simulink model "S250205simul_switch_2023a"  (R2024b)
settings: Solver=FixedStepDiscrete  StartTime=0  StopTime=60  FixedStep=0.01  RelTol=1e-3  AbsTol=1e-6
undefined symbols (not defined in the file or in its folder): a, b, c, d, f, g, switch_logic, VmcRgn_C_C, VmcRgn_J_C, VmcRgn_k_1to2_C, VmcRgn_k_2to3_C, VmcRgn_k_2to6_C, VmcRgn_k_3to4_C, VmcRgn_k_5to2_C, VmcRgn_k_6to2_C, VmcRgn_Kp_C, VmcRgn_L_C, VmcRgn_lf_C, VmcRgn_lr_C, VmcRgn_mass_C, VmcRgn_Mot2Whl_C, VmcRgn_PedDep_thrs_C, VmcRgn_phs2_k_C, VmcRgn_phs2_tq_C, VmcRgn_phs3_tq_C, VmcRgn_phs4_tq_C, VmcRgn_phs5_tq_C, VmcRgn_phs6_tq_C, VmcRgn_r_e_C, VmcRgn_R_whl_C, VmcRgn_SAS_thrs_C, VmcRgn_slip_max_C, VmcRgn_slip_max_gain_F_C, VmcRgn_slip_max_gain_R_C, VmcRgn_sup_tq_C, VmcRgn_t_pred_C, VmcRgn_target_w_acc_C, VmcRgn_tTs, VmcRgn_tTsinMs_C, VmcRgn_Yaw_thrs_C, yaw_flag
libraries: simulink x26, simulink_need_slupdate x1
(part 3 of 3)

== system S250205simul_switch_2023a/SlipCtrlFL/DiscreteDerivative ==
  note: U(k)
  note: ( U(k) - U(k-1) )
  U : Inport
  Constant : Constant  Value=Ts  OutDataTypeStr=uint16
  Data Type Conversion : DataTypeConversion  OutDataTypeStr=single  SaturateOnIntegerOverflow=off  RndMeth=Floor
  Data Type Conversion1 : DataTypeConversion  OutDataTypeStr=single  SaturateOnIntegerOverflow=off  RndMeth=Floor
  Data Type Conversion2 : DataTypeConversion  RndMeth=Round  LockScale=on
  Diff : Sum  Description=Add in CPU  Inputs=+-  OutDataTypeStr=single  AccumDataTypeStr=single  SaturateOnIntegerOverflow=on
  Divide : Product  Inputs=*/  OutDataTypeStr=single
  UD : UnitDelay  Description=Store in Global RAM  DisableCoverage=on  SampleTime=-1  HasFrameUpgradeWarning=on
  ms-to-s : Gain  Gain=0.001  ParamDataTypeStr=single  OutDataTypeStr=single
  Y : Outport  OutDataTypeStr=out_type  InitialOutput=0  VectorParamsAs1DForOutWhenUnconnected=off
  wires:
  Constant/1 -> Data Type Conversion1/1
  Divide/1 -> Diff/1, UD/1
  Diff/1 -> Data Type Conversion2/1
  UD/1 -> Diff/2  "U(k-1)"
  U/1 -> Data Type Conversion/1
  Data Type Conversion/1 -> Divide/1
  Data Type Conversion1/1 -> ms-to-s/1
  ms-to-s/1 -> Divide/2
  Data Type Conversion2/1 -> Y/1

== system S250205simul_switch_2023a/SlipCtrlFL/Sat_-1to1 ==
  In1 : Inport
  Constant : Constant  Value=-1  OutDataTypeStr=single
  Constant1 : Constant  OutDataTypeStr=single
  Switch1 : Switch  Criteria=u2 > Threshold  Threshold=1  SaturateOnIntegerOverflow=off  InputSameDT=off
  Switch4 : Switch  Criteria=u2 > Threshold  Threshold=-1  SaturateOnIntegerOverflow=off  InputSameDT=off
  Out1 : Outport
  wires:
  In1/1 -> Switch4/1, Switch4/2
  Switch4/1 -> Switch1/3, Switch1/2
  Constant/1 -> Switch4/3
  Constant1/1 -> Switch1/1
  Switch1/1 -> Out1/1

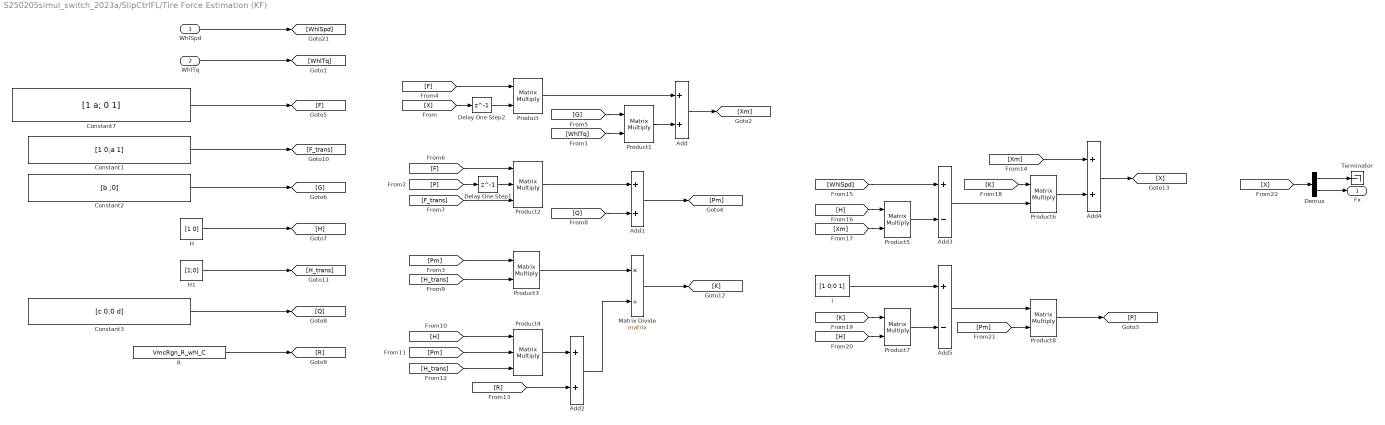
== system S250205simul_switch_2023a/SlipCtrlFL/Tire Force Estimation (KF) ==
  WhlSpd : Inport
  WhlTq : Inport  Port=2
  Add : Sum  OutDataTypeStr=single
  Add1 : Sum  OutDataTypeStr=single
  Add2 : Sum
  Add3 : Sum  Inputs=+-  OutDataTypeStr=single
  Add4 : Sum  OutDataTypeStr=single
  Add5 : Sum  Inputs=+-  OutDataTypeStr=single
  Constant1 : Constant  Value=[1 0;a 1]  VectorParams1D=off  SampleTime=-1  LockScale=on  mask(Customized constant block){}
      settings: AttributesFormatString=OutType: %<OutDataTypeStr>
  Constant2 : Constant  Value=[b ;0]  VectorParams1D=off  SampleTime=-1  LockScale=on  mask(Customized constant block){}
      settings: AttributesFormatString=OutType: %<OutDataTypeStr>
  Constant3 : Constant  Value=[c 0;0 d]  VectorParams1D=off  SampleTime=-1  LockScale=on  mask(Customized constant block){}
      settings: AttributesFormatString=OutType: %<OutDataTypeStr>
  Constant7 : Constant  Value=[1 a; 0 1]  VectorParams1D=off  SampleTime=-1  LockScale=on  mask(Customized constant block){}
      settings: AttributesFormatString=OutType: %<OutDataTypeStr>
  Delay One Step1 : Delay  DelayLength=1  InitialCondition=diag([64.1 0])
  Delay One Step2 : Delay  DelayLength=1  InitialCondition=[64.1; 0]
  Demux : Demux  Outputs=2
  H : Constant  Value=[1 0]  VectorParams1D=off  OutDataTypeStr=single  SampleTime=-1
  H1 : Constant  Value=[1;0]  VectorParams1D=off  OutDataTypeStr=single  SampleTime=-1
  I : Constant  Value=[1 0;0 1]  VectorParams1D=off  OutDataTypeStr=single  SampleTime=-1
  Matrix Divide : Product  Inputs=*/  Multiplication=Matrix(*)  OutDataTypeStr=single
  Product{,1,3,5..8} (7 alike) : Product  Multiplication=Matrix(*)
  Product2 : Product  Inputs=3  Multiplication=Matrix(*)
  Product4 : Product  Inputs=3  Multiplication=Matrix(*)
  R : Constant  Value=VmcRgn_R_whl_C  VectorParams1D=off  OutDataTypeStr=single  SampleTime=-1
  Terminator : Terminator
  Fx : Outport
  wires:
  WhlSpd/1 -> [WhlSpd]
  WhlTq/1 -> [WhlTq]
  [F] -> Product/1
  Product/1 -> Add/1
  [G] -> Product1/1
  [WhlTq] -> Product1/2
  Product1/1 -> Add/2
  Add/1 -> [Xm]
  [P] -> Delay One Step1/1
  Delay One Step1/1 -> Product2/2
  [F_trans] -> Product2/3
  Add1/1 -> [Pm]
  [Pm] -> Product3/1
  Constant7/1 -> [F]
  Constant2/1 -> [G]
  H/1 -> [H]
  Constant3/1 -> [Q]
  R/1 -> [R]
  [F] -> Product2/1
  Constant1/1 -> [F_trans]
  H1/1 -> [H_trans]
  Product2/1 -> Add1/1
  [Q] -> Add1/2
  [H_trans] -> Product3/2
  [H] -> Product4/1
  [H_trans] -> Product4/3
  [Pm] -> Product4/2
  Product4/1 -> Add2/1
  [R] -> Add2/2
  Product3/1 -> Matrix Divide/1
  Add2/1 -> Matrix Divide/2
  Matrix Divide/1 -> [K]
  [WhlSpd] -> Add3/1
  Product5/1 -> Add3/2
  [H] -> Product5/1
  [Xm] -> Product5/2
  Add3/1 -> Product6/2
  [K] -> Product6/1
  Product6/1 -> Add4/2
  [Xm] -> Add4/1
  Add4/1 -> [X]
  I/1 -> Add5/1
  [K] -> Product7/1
  [H] -> Product7/2
  Product7/1 -> Add5/2
  Add5/1 -> Product8/1
  [Pm] -> Product8/2
  Product8/1 -> [P]
  Delay One Step2/1 -> Product/2
  [X] -> Delay One Step2/1
  Demux/2 -> Fx/1
  Demux/1 -> Terminator/1
  [X] -> Demux/1

== system S250205simul_switch_2023a/SlipCtrlFL/Triggered Subsystem ==
  In1 : Inport
  Trigger : TriggerPort  VariantControl=(inherit)
  Out1 : Outport
  wires:
  In1/1 -> Out1/1

== system S250205simul_switch_2023a/SlipCtrlFR/DiscreteDerivative ==
  note: U(k)
  note: ( U(k) - U(k-1) )
  U : Inport
  Constant : Constant  Value=Ts  OutDataTypeStr=uint16
  Data Type Conversion : DataTypeConversion  OutDataTypeStr=single  SaturateOnIntegerOverflow=off  RndMeth=Floor
  Data Type Conversion1 : DataTypeConversion  OutDataTypeStr=single  SaturateOnIntegerOverflow=off  RndMeth=Floor
  Data Type Conversion2 : DataTypeConversion  RndMeth=Round  LockScale=on
  Diff : Sum  Description=Add in CPU  Inputs=+-  OutDataTypeStr=single  AccumDataTypeStr=single  SaturateOnIntegerOverflow=on
  Divide : Product  Inputs=*/  OutDataTypeStr=single
  UD : UnitDelay  Description=Store in Global RAM  DisableCoverage=on  SampleTime=-1  HasFrameUpgradeWarning=on
  ms-to-s : Gain  Gain=0.001  ParamDataTypeStr=single  OutDataTypeStr=single
  Y : Outport  OutDataTypeStr=out_type  InitialOutput=0  VectorParamsAs1DForOutWhenUnconnected=off
  wires:
  Constant/1 -> Data Type Conversion1/1
  Divide/1 -> Diff/1, UD/1
  Diff/1 -> Data Type Conversion2/1
  UD/1 -> Diff/2  "U(k-1)"
  U/1 -> Data Type Conversion/1
  Data Type Conversion/1 -> Divide/1
  Data Type Conversion1/1 -> ms-to-s/1
  ms-to-s/1 -> Divide/2
  Data Type Conversion2/1 -> Y/1

== system S250205simul_switch_2023a/SlipCtrlFR/Sat_-1to1 ==
  In1 : Inport
  Constant : Constant  Value=-1  OutDataTypeStr=single
  Constant1 : Constant  OutDataTypeStr=single
  Switch1 : Switch  Criteria=u2 > Threshold  Threshold=1  SaturateOnIntegerOverflow=off  InputSameDT=off
  Switch4 : Switch  Criteria=u2 > Threshold  Threshold=-1  SaturateOnIntegerOverflow=off  InputSameDT=off
  Out1 : Outport
  wires:
  In1/1 -> Switch4/1, Switch4/2
  Switch4/1 -> Switch1/3, Switch1/2
  Constant/1 -> Switch4/3
  Constant1/1 -> Switch1/1
  Switch1/1 -> Out1/1

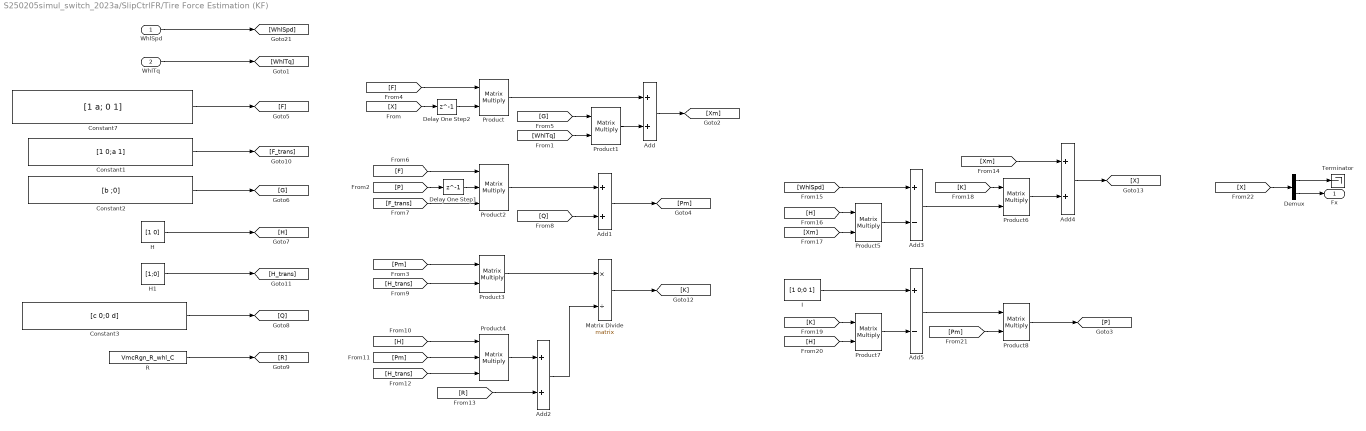
== system S250205simul_switch_2023a/SlipCtrlFR/Tire Force Estimation (KF) ==
  WhlSpd : Inport
  WhlTq : Inport  Port=2
  Add : Sum  OutDataTypeStr=single
  Add1 : Sum  OutDataTypeStr=single
  Add2 : Sum
  Add3 : Sum  Inputs=+-  OutDataTypeStr=single
  Add4 : Sum  OutDataTypeStr=single
  Add5 : Sum  Inputs=+-  OutDataTypeStr=single
  Constant1 : Constant  Value=[1 0;a 1]  VectorParams1D=off  SampleTime=-1  LockScale=on  mask(Customized constant block){}
      settings: AttributesFormatString=OutType: %<OutDataTypeStr>
  Constant2 : Constant  Value=[b ;0]  VectorParams1D=off  SampleTime=-1  LockScale=on  mask(Customized constant block){}
      settings: AttributesFormatString=OutType: %<OutDataTypeStr>
  Constant3 : Constant  Value=[c 0;0 d]  VectorParams1D=off  SampleTime=-1  LockScale=on  mask(Customized constant block){}
      settings: AttributesFormatString=OutType: %<OutDataTypeStr>
  Constant7 : Constant  Value=[1 a; 0 1]  VectorParams1D=off  SampleTime=-1  LockScale=on  mask(Customized constant block){}
      settings: AttributesFormatString=OutType: %<OutDataTypeStr>
  Delay One Step1 : Delay  DelayLength=1  InitialCondition=diag([64.1 0])
  Delay One Step2 : Delay  DelayLength=1  InitialCondition=[64.1; 0]
  Demux : Demux  Outputs=2
  H : Constant  Value=[1 0]  VectorParams1D=off  OutDataTypeStr=single  SampleTime=-1
  H1 : Constant  Value=[1;0]  VectorParams1D=off  OutDataTypeStr=single  SampleTime=-1
  I : Constant  Value=[1 0;0 1]  VectorParams1D=off  OutDataTypeStr=single  SampleTime=-1
  Matrix Divide : Product  Inputs=*/  Multiplication=Matrix(*)  OutDataTypeStr=single
  Product{,1,3,5..8} (7 alike) : Product  Multiplication=Matrix(*)
  Product2 : Product  Inputs=3  Multiplication=Matrix(*)
  Product4 : Product  Inputs=3  Multiplication=Matrix(*)
  R : Constant  Value=VmcRgn_R_whl_C  OutDataTypeStr=single  SampleTime=-1
  Terminator : Terminator
  Fx : Outport
  wires:
  WhlSpd/1 -> [WhlSpd]
  WhlTq/1 -> [WhlTq]
  [F] -> Product/1
  Product/1 -> Add/1
  [G] -> Product1/1
  [WhlTq] -> Product1/2
  Product1/1 -> Add/2
  Add/1 -> [Xm]
  [P] -> Delay One Step1/1
  Delay One Step1/1 -> Product2/2
  [F_trans] -> Product2/3
  Add1/1 -> [Pm]
  [Pm] -> Product3/1
  Constant7/1 -> [F]
  Constant2/1 -> [G]
  H/1 -> [H]
  Constant3/1 -> [Q]
  R/1 -> [R]
  [F] -> Product2/1
  Constant1/1 -> [F_trans]
  H1/1 -> [H_trans]
  Product2/1 -> Add1/1
  [Q] -> Add1/2
  [H_trans] -> Product3/2
  [H] -> Product4/1
  [H_trans] -> Product4/3
  [Pm] -> Product4/2
  Product4/1 -> Add2/1
  [R] -> Add2/2
  Product3/1 -> Matrix Divide/1
  Add2/1 -> Matrix Divide/2
  Matrix Divide/1 -> [K]
  [WhlSpd] -> Add3/1
  Product5/1 -> Add3/2
  [H] -> Product5/1
  [Xm] -> Product5/2
  Add3/1 -> Product6/2
  [K] -> Product6/1
  Product6/1 -> Add4/2
  [Xm] -> Add4/1
  Add4/1 -> [X]
  I/1 -> Add5/1
  [K] -> Product7/1
  [H] -> Product7/2
  Product7/1 -> Add5/2
  Add5/1 -> Product8/1
  [Pm] -> Product8/2
  Product8/1 -> [P]
  Delay One Step2/1 -> Product/2
  [X] -> Delay One Step2/1
  Demux/2 -> Fx/1
  Demux/1 -> Terminator/1
  [X] -> Demux/1

== system S250205simul_switch_2023a/SlipCtrlFR/Triggered Subsystem ==
  In1 : Inport
  Trigger : TriggerPort  VariantControl=(inherit)
  Out1 : Outport
  wires:
  In1/1 -> Out1/1

== system S250205simul_switch_2023a/SlipCtrlRL/DiscreteDerivative ==
  note: U(k)
  note: ( U(k) - U(k-1) )
  U : Inport
  Constant : Constant  Value=Ts  OutDataTypeStr=uint16
  Data Type Conversion : DataTypeConversion  OutDataTypeStr=single  SaturateOnIntegerOverflow=off  RndMeth=Floor
  Data Type Conversion1 : DataTypeConversion  OutDataTypeStr=single  SaturateOnIntegerOverflow=off  RndMeth=Floor
  Data Type Conversion2 : DataTypeConversion  RndMeth=Round  LockScale=on
  Diff : Sum  Description=Add in CPU  Inputs=+-  OutDataTypeStr=single  AccumDataTypeStr=single  SaturateOnIntegerOverflow=on
  Divide : Product  Inputs=*/  OutDataTypeStr=single
  UD : UnitDelay  Description=Store in Global RAM  DisableCoverage=on  SampleTime=-1  HasFrameUpgradeWarning=on
  ms-to-s : Gain  Gain=0.001  ParamDataTypeStr=single  OutDataTypeStr=single
  Y : Outport  OutDataTypeStr=out_type  InitialOutput=0  VectorParamsAs1DForOutWhenUnconnected=off
  wires:
  Constant/1 -> Data Type Conversion1/1
  Divide/1 -> Diff/1, UD/1
  Diff/1 -> Data Type Conversion2/1
  UD/1 -> Diff/2  "U(k-1)"
  U/1 -> Data Type Conversion/1
  Data Type Conversion/1 -> Divide/1
  Data Type Conversion1/1 -> ms-to-s/1
  ms-to-s/1 -> Divide/2
  Data Type Conversion2/1 -> Y/1

== system S250205simul_switch_2023a/SlipCtrlRL/Sat_-1to1 ==
  In1 : Inport
  Constant : Constant  Value=-1  OutDataTypeStr=single
  Constant1 : Constant  OutDataTypeStr=single
  Switch1 : Switch  Criteria=u2 > Threshold  Threshold=1  SaturateOnIntegerOverflow=off  InputSameDT=off
  Switch4 : Switch  Criteria=u2 > Threshold  Threshold=-1  SaturateOnIntegerOverflow=off  InputSameDT=off
  Out1 : Outport
  wires:
  In1/1 -> Switch4/1, Switch4/2
  Switch4/1 -> Switch1/3, Switch1/2
  Constant/1 -> Switch4/3
  Constant1/1 -> Switch1/1
  Switch1/1 -> Out1/1

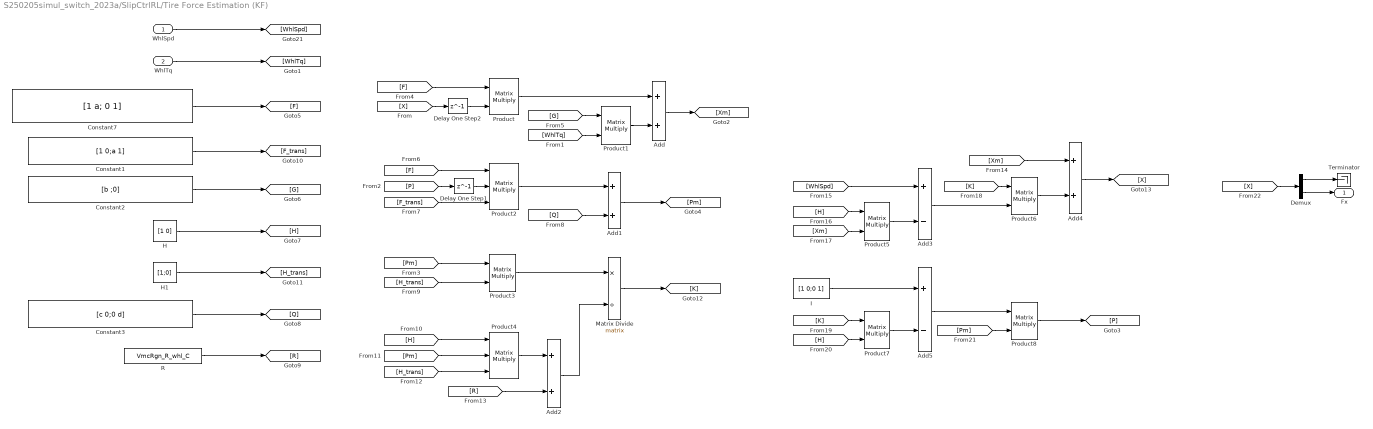
== system S250205simul_switch_2023a/SlipCtrlRL/Tire Force Estimation (KF) ==
  WhlSpd : Inport
  WhlTq : Inport  Port=2
  Add{,1..2,4} (4 alike) : Sum  OutDataTypeStr=single
  Add3 : Sum  Inputs=+-  OutDataTypeStr=single
  Add5 : Sum  Inputs=+-  OutDataTypeStr=single
  Constant1 : Constant  Value=[1 0;a 1]  VectorParams1D=off  SampleTime=-1  LockScale=on  mask(Customized constant block){}
      settings: AttributesFormatString=OutType: %<OutDataTypeStr>
  Constant2 : Constant  Value=[b ;0]  VectorParams1D=off  SampleTime=-1  LockScale=on  mask(Customized constant block){}
      settings: AttributesFormatString=OutType: %<OutDataTypeStr>
  Constant3 : Constant  Value=[c 0;0 d]  VectorParams1D=off  SampleTime=-1  LockScale=on  mask(Customized constant block){}
      settings: AttributesFormatString=OutType: %<OutDataTypeStr>
  Constant7 : Constant  Value=[1 a; 0 1]  VectorParams1D=off  SampleTime=-1  LockScale=on  mask(Customized constant block){}
      settings: AttributesFormatString=OutType: %<OutDataTypeStr>
  Delay One Step1 : Delay  DelayLength=1  InitialCondition=diag([64.1 0])
  Delay One Step2 : Delay  DelayLength=1  InitialCondition=[64.1; 0]
  Demux : Demux  Outputs=2
  H : Constant  Value=[1 0]  VectorParams1D=off  OutDataTypeStr=single  SampleTime=-1
  H1 : Constant  Value=[1;0]  VectorParams1D=off  OutDataTypeStr=single  SampleTime=-1
  I : Constant  Value=[1 0;0 1]  VectorParams1D=off  OutDataTypeStr=single  SampleTime=-1
  Matrix Divide : Product  Inputs=*/  Multiplication=Matrix(*)  OutDataTypeStr=single
  Product{,1,3,5..8} (7 alike) : Product  Multiplication=Matrix(*)
  Product2 : Product  Inputs=3  Multiplication=Matrix(*)
  Product4 : Product  Inputs=3  Multiplication=Matrix(*)
  R : Constant  Value=VmcRgn_R_whl_C  OutDataTypeStr=single  SampleTime=-1
  Terminator : Terminator
  Fx : Outport
  wires:
  WhlSpd/1 -> [WhlSpd]
  WhlTq/1 -> [WhlTq]
  [F] -> Product/1
  Product/1 -> Add/1
  [G] -> Product1/1
  [WhlTq] -> Product1/2
  Product1/1 -> Add/2
  Add/1 -> [Xm]
  [P] -> Delay One Step1/1
  Delay One Step1/1 -> Product2/2
  [F_trans] -> Product2/3
  Add1/1 -> [Pm]
  [Pm] -> Product3/1
  Constant7/1 -> [F]
  Constant2/1 -> [G]
  H/1 -> [H]
  Constant3/1 -> [Q]
  R/1 -> [R]
  [F] -> Product2/1
  Constant1/1 -> [F_trans]
  H1/1 -> [H_trans]
  Product2/1 -> Add1/1
  [Q] -> Add1/2
  [H_trans] -> Product3/2
  [H] -> Product4/1
  [H_trans] -> Product4/3
  [Pm] -> Product4/2
  Product4/1 -> Add2/1
  [R] -> Add2/2
  Product3/1 -> Matrix Divide/1
  Add2/1 -> Matrix Divide/2
  Matrix Divide/1 -> [K]
  [WhlSpd] -> Add3/1
  Product5/1 -> Add3/2
  [H] -> Product5/1
  [Xm] -> Product5/2
  Add3/1 -> Product6/2
  [K] -> Product6/1
  Product6/1 -> Add4/2
  [Xm] -> Add4/1
  Add4/1 -> [X]
  I/1 -> Add5/1
  [K] -> Product7/1
  [H] -> Product7/2
  Product7/1 -> Add5/2
  Add5/1 -> Product8/1
  [Pm] -> Product8/2
  Product8/1 -> [P]
  Delay One Step2/1 -> Product/2
  [X] -> Delay One Step2/1
  [X] -> Demux/1
  Demux/2 -> Fx/1
  Demux/1 -> Terminator/1

== system S250205simul_switch_2023a/SlipCtrlRL/Triggered Subsystem ==
  In1 : Inport
  Trigger : TriggerPort  VariantControl=(inherit)
  Out1 : Outport
  wires:
  In1/1 -> Out1/1

== system S250205simul_switch_2023a/SlipCtrlRL/Triggered Subsystem1 ==
  In1 : Inport
  Trigger : TriggerPort  VariantControl=(inherit)
  Out1 : Outport
  wires:
  In1/1 -> Out1/1

== system S250205simul_switch_2023a/SlipCtrlRR/DiscreteDerivative ==
  note: U(k)
  note: ( U(k) - U(k-1) )
  U : Inport
  Constant : Constant  Value=Ts  OutDataTypeStr=uint16
  Data Type Conversion : DataTypeConversion  OutDataTypeStr=single  SaturateOnIntegerOverflow=off  RndMeth=Floor
  Data Type Conversion1 : DataTypeConversion  OutDataTypeStr=single  SaturateOnIntegerOverflow=off  RndMeth=Floor
  Data Type Conversion2 : DataTypeConversion  RndMeth=Round  LockScale=on
  Diff : Sum  Description=Add in CPU  Inputs=+-  OutDataTypeStr=single  AccumDataTypeStr=single  SaturateOnIntegerOverflow=on
  Divide : Product  Inputs=*/  OutDataTypeStr=single
  UD : UnitDelay  Description=Store in Global RAM  DisableCoverage=on  SampleTime=-1  HasFrameUpgradeWarning=on
  ms-to-s : Gain  Gain=0.001  ParamDataTypeStr=single  OutDataTypeStr=single
  Y : Outport  OutDataTypeStr=out_type  InitialOutput=0  VectorParamsAs1DForOutWhenUnconnected=off
  wires:
  Constant/1 -> Data Type Conversion1/1
  Divide/1 -> Diff/1, UD/1
  Diff/1 -> Data Type Conversion2/1
  UD/1 -> Diff/2  "U(k-1)"
  U/1 -> Data Type Conversion/1
  Data Type Conversion/1 -> Divide/1
  Data Type Conversion1/1 -> ms-to-s/1
  ms-to-s/1 -> Divide/2
  Data Type Conversion2/1 -> Y/1

== system S250205simul_switch_2023a/SlipCtrlRR/Sat_-1to1 ==
  In1 : Inport
  Constant : Constant  Value=-1  OutDataTypeStr=single
  Constant1 : Constant  OutDataTypeStr=single
  Switch1 : Switch  Criteria=u2 > Threshold  Threshold=1  SaturateOnIntegerOverflow=off  InputSameDT=off
  Switch4 : Switch  Criteria=u2 > Threshold  Threshold=-1  SaturateOnIntegerOverflow=off  InputSameDT=off
  Out1 : Outport
  wires:
  In1/1 -> Switch4/1, Switch4/2
  Switch4/1 -> Switch1/3, Switch1/2
  Constant/1 -> Switch4/3
  Constant1/1 -> Switch1/1
  Switch1/1 -> Out1/1

== system S250205simul_switch_2023a/SlipCtrlRR/Tire Force Estimation (KF) ==
  WhlSpd : Inport
  WhlTq : Inport  Port=2
  Add{,1..2,4} (4 alike) : Sum  OutDataTypeStr=single
  Add3 : Sum  Inputs=+-  OutDataTypeStr=single
  Add5 : Sum  Inputs=+-  OutDataTypeStr=single
  Constant1 : Constant  Value=[1 0;a 1]  VectorParams1D=off  SampleTime=-1  LockScale=on  mask(Customized constant block){}
      settings: AttributesFormatString=OutType: %<OutDataTypeStr>
  Constant2 : Constant  Value=[b ;0]  VectorParams1D=off  SampleTime=-1  LockScale=on  mask(Customized constant block){}
      settings: AttributesFormatString=OutType: %<OutDataTypeStr>
  Constant3 : Constant  Value=[c 0;0 d]  VectorParams1D=off  SampleTime=-1  LockScale=on  mask(Customized constant block){}
      settings: AttributesFormatString=OutType: %<OutDataTypeStr>
  Constant7 : Constant  Value=[1 a; 0 1]  VectorParams1D=off  SampleTime=-1  LockScale=on  mask(Customized constant block){}
      settings: AttributesFormatString=OutType: %<OutDataTypeStr>
  Delay One Step1 : Delay  DelayLength=1  InitialCondition=diag([64.1 0])
  Delay One Step2 : Delay  DelayLength=1  InitialCondition=[64.1; 0]
  Demux : Demux  Outputs=2
  H : Constant  Value=[1 0]  VectorParams1D=off  OutDataTypeStr=single  SampleTime=-1
  H1 : Constant  Value=[1;0]  VectorParams1D=off  OutDataTypeStr=single  SampleTime=-1
  I : Constant  Value=[1 0;0 1]  VectorParams1D=off  OutDataTypeStr=single  SampleTime=-1
  Matrix Divide : Product  Inputs=*/  Multiplication=Matrix(*)  OutDataTypeStr=single
  Product{,1,3,5..8} (7 alike) : Product  Multiplication=Matrix(*)
  Product2 : Product  Inputs=3  Multiplication=Matrix(*)
  Product4 : Product  Inputs=3  Multiplication=Matrix(*)
  R : Constant  Value=VmcRgn_R_whl_C  OutDataTypeStr=single  SampleTime=-1
  Terminator : Terminator
  Fx : Outport
  wires:
  WhlSpd/1 -> [WhlSpd]
  WhlTq/1 -> [WhlTq]
  [F] -> Product/1
  Product/1 -> Add/1
  [G] -> Product1/1
  [WhlTq] -> Product1/2
  Product1/1 -> Add/2
  Add/1 -> [Xm]
  [P] -> Delay One Step1/1
  Delay One Step1/1 -> Product2/2
  [F_trans] -> Product2/3
  Add1/1 -> [Pm]
  [Pm] -> Product3/1
  Constant7/1 -> [F]
  Constant2/1 -> [G]
  H/1 -> [H]
  Constant3/1 -> [Q]
  R/1 -> [R]
  [F] -> Product2/1
  Constant1/1 -> [F_trans]
  H1/1 -> [H_trans]
  Product2/1 -> Add1/1
  [Q] -> Add1/2
  [H_trans] -> Product3/2
  [H] -> Product4/1
  [H_trans] -> Product4/3
  [Pm] -> Product4/2
  Product4/1 -> Add2/1
  [R] -> Add2/2
  Product3/1 -> Matrix Divide/1
  Add2/1 -> Matrix Divide/2
  Matrix Divide/1 -> [K]
  [WhlSpd] -> Add3/1
  Product5/1 -> Add3/2
  [H] -> Product5/1
  [Xm] -> Product5/2
  Add3/1 -> Product6/2
  [K] -> Product6/1
  Product6/1 -> Add4/2
  [Xm] -> Add4/1
  Add4/1 -> [X]
  I/1 -> Add5/1
  [K] -> Product7/1
  [H] -> Product7/2
  Product7/1 -> Add5/2
  Add5/1 -> Product8/1
  [Pm] -> Product8/2
  Product8/1 -> [P]
  Delay One Step2/1 -> Product/2
  [X] -> Delay One Step2/1
  Demux/2 -> Fx/1
  Demux/1 -> Terminator/1
  [X] -> Demux/1

== system S250205simul_switch_2023a/SlipCtrlRR/Triggered Subsystem ==
  In1 : Inport
  Trigger : TriggerPort  VariantControl=(inherit)
  Out1 : Outport
  wires:
  In1/1 -> Out1/1

== system S250205simul_switch_2023a/Torque/Rate Limiter4 ==
  In : Inport
  Add : Sum  Inputs=-+
  Add1 : Sum
  Add2 : Sum
  Delay One Step : Delay  DelayLength=1
  Lower Bound : Constant  Value=-3000  OutDataTypeStr=single
  Product : Product
  Product1 : Product
  Relational Operator : RelationalOperator  OutDataTypeStr=boolean  RndMeth=Simplest  InputSameDT=off
  Relational Operator1 : RelationalOperator  OutDataTypeStr=boolean  RndMeth=Simplest  InputSameDT=off
  Switch : Switch  Criteria=u2 > Threshold  SaturateOnIntegerOverflow=off  InputSameDT=off
  Switch1 : Switch  Criteria=u2 > Threshold  SaturateOnIntegerOverflow=off  InputSameDT=off
  Ts : Constant  Value=VmcRgn_tTs  OutDataTypeStr=single
  Upper Bound : Constant  Value=3000  OutDataTypeStr=single
  Out : Outport
  wires:
  In/1 -> Switch/1, Add/2
  Add/1 -> Relational Operator1/1, Relational Operator/1
  Relational Operator/1 -> Switch/2
  Product/1 -> Add2/1, Relational Operator/2
  Ts/1 -> [Ts]
  [Ts] -> Product1/2
  [Ts] -> Product/2
  Upper Bound/1 -> [ub]
  Lower Bound/1 -> [lb]
  [ub] -> Product1/1
  [lb] -> Product/1
  Product1/1 -> Relational Operator1/2, Add1/2
  Relational Operator1/1 -> Switch1/2
  Add1/1 -> Switch1/1
  Switch/1 -> Switch1/3
  Switch1/1 -> Delay One Step/1, Out/1
  Delay One Step/1 -> Add1/1, Add2/2, Add/1
  Add2/1 -> Switch/3

== system S250205simul_switch_2023a/Yaw Stability Control1/DiscreteIntegrator_ExtRst2 ==
  note: ( Ts * U(k) + U(k-1) )
  U : Inport
  Rst : Inport  Port=2  OutDataTypeStr=boolean
  Accumulator : Sum  Description=Add in CPU  OutDataTypeStr=single  AccumDataTypeStr=single  SaturateOnIntegerOverflow=on
  Constant : Constant  Value=Ts  OutDataTypeStr=uint16
  Constant1 : Constant  Value=0  OutDataTypeStr=single
  Data Type Conversion : DataTypeConversion  OutDataTypeStr=single  SaturateOnIntegerOverflow=off  RndMeth=Floor
  Data Type Conversion1 : DataTypeConversion  OutDataTypeStr=single  SaturateOnIntegerOverflow=off  RndMeth=Floor
  Data Type Conversion2 : DataTypeConversion  RndMeth=Round  LockScale=on
  Divide : Product  Inputs=**  OutDataTypeStr=single
  Switch : Switch  Criteria=u2 ~= 0  SaturateOnIntegerOverflow=off  InputSameDT=off
  Unit Delay Resettable : simulink_need_slupdate/Unit Delay Resettable  vinit=0.0  tsamp=-1
  ms-to-s : Gain  Gain=0.001  ParamDataTypeStr=single  OutDataTypeStr=single
  Y : Outport  OutDataTypeStr=out_type  InitialOutput=0  VectorParamsAs1DForOutWhenUnconnected=off
  wires:
  Data Type Conversion2/1 -> Y/1
  Rst/1 -> Unit Delay Resettable/2, Switch/2
  Unit Delay Resettable/1 -> Accumulator/1  "U(k-1)"
  Constant/1 -> Data Type Conversion1/1
  Accumulator/1 -> Data Type Conversion2/1, Unit Delay Resettable/1
  U/1 -> Data Type Conversion/1
  Data Type Conversion1/1 -> ms-to-s/1
  ms-to-s/1 -> Divide/2
  Data Type Conversion/1 -> Divide/1
  Divide/1 -> Switch/3
  Constant1/1 -> Switch/1
  Switch/1 -> Accumulator/2

== system S250205simul_switch_2023a/Yaw Stability Control1/Rate Limiter ==
  In : Inport
  Add : Sum  Inputs=-+
  Add1 : Sum  OutDataTypeStr=single
  Add2 : Sum
  Delay One Step : Delay  DelayLength=1
  Lower Bound : Constant  Value=-3000
  Product : Product
  Product1 : Product  OutDataTypeStr=single
  Relational Operator : RelationalOperator  OutDataTypeStr=boolean  RndMeth=Simplest  InputSameDT=off
  Relational Operator1 : RelationalOperator  OutDataTypeStr=boolean  RndMeth=Simplest  InputSameDT=off
  Switch : Switch  Criteria=u2 > Threshold  SaturateOnIntegerOverflow=off  InputSameDT=off
  Switch1 : Switch  Criteria=u2 > Threshold  OutDataTypeStr=single  SaturateOnIntegerOverflow=off  InputSameDT=off
  Ts : Constant  Value=VmcRgn_tTs
  Upper Bound : Constant  Value=3000
  Out : Outport
  wires:
  In/1 -> Switch/1, Add/2
  Add/1 -> Relational Operator1/1, Relational Operator/1
  Relational Operator/1 -> Switch/2
  Product/1 -> Add2/1, Relational Operator/2
  Ts/1 -> [Ts]
  [Ts] -> Product1/2
  [Ts] -> Product/2
  Upper Bound/1 -> [ub]
  Lower Bound/1 -> [lb]
  [ub] -> Product1/1
  [lb] -> Product/1
  Product1/1 -> Relational Operator1/2, Add1/2
  Relational Operator1/1 -> Switch1/2
  Add1/1 -> Switch1/1
  Switch/1 -> Switch1/3
  Switch1/1 -> Delay One Step/1, Out/1
  Delay One Step/1 -> Add1/1, Add2/2, Add/1
  Add2/1 -> Switch/3

== system S250205simul_switch_2023a/Yaw Stability Control1/Rate Limiter1 ==
  In : Inport
  Add : Sum  Inputs=-+
  Add1 : Sum
  Add2 : Sum
  Delay One Step : Delay  DelayLength=1
  Lower Bound : Constant  Value=-3000
  Product : Product
  Product1 : Product
  Relational Operator : RelationalOperator  OutDataTypeStr=boolean  RndMeth=Simplest  InputSameDT=off
  Relational Operator1 : RelationalOperator  OutDataTypeStr=boolean  RndMeth=Simplest  InputSameDT=off
  Switch : Switch  Criteria=u2 > Threshold  SaturateOnIntegerOverflow=off  InputSameDT=off
  Switch1 : Switch  Criteria=u2 > Threshold  SaturateOnIntegerOverflow=off  InputSameDT=off
  Ts : Constant  Value=VmcRgn_tTs
  Upper Bound : Constant  Value=3000
  Out : Outport
  wires:
  In/1 -> Switch/1, Add/2
  Add/1 -> Relational Operator1/1, Relational Operator/1
  Relational Operator/1 -> Switch/2
  Product/1 -> Add2/1, Relational Operator/2
  Ts/1 -> [Ts]
  [Ts] -> Product1/2
  [Ts] -> Product/2
  Upper Bound/1 -> [ub]
  Lower Bound/1 -> [lb]
  [ub] -> Product1/1
  [lb] -> Product/1
  Product1/1 -> Relational Operator1/2, Add1/2
  Relational Operator1/1 -> Switch1/2
  Add1/1 -> Switch1/1
  Switch/1 -> Switch1/3
  Switch1/1 -> Delay One Step/1, Out/1
  Delay One Step/1 -> Add1/1, Add2/2, Add/1
  Add2/1 -> Switch/3

== stateflow chart S250205simul_switch_2023a/Slip Control State1/Slip_Stateflow ==
  state Coasting
    state State0
      en, du: state = 0;
    state State1
      en, du:
      state = 1;
    state State2
      en, du:
      state = 2;
    state State3
      en, du:
      state = 3;
    state State4
      en, du:
      state = 4;
    (default) -> State0
    State0 -> State1 : [(ph_FL==1)|(ph_FR==1)|(ph_RL==1)|(ph_RR==1)]
    State1 -> State2 [order 1] : [(ph_FL>=2)|(ph_FR>=2)]
    State2 -> State1 [order 1] : [(ph_FL<=1)&(ph_FR<=1)]
    State3 -> State1 [order 1] : [(ph_RL<=1)&(ph_RR<=1)]
    State1 -> State3 [order 2] : [(ph_RL>=2)|(ph_RR>=2)]
    State4 -> State2 [order 1] : [(ph_RL==1)&(ph_RR==1)]
    State2 -> State4 [order 2] : [(ph_RL>=2)|(ph_RR>=2)]
    State3 -> State4 [order 2] : [(ph_FL>=2)|(ph_FR>=2)]
    State4 -> State3 [order 2] : [(ph_FL<=1)&(ph_FR<=1)]
  state drive
    en, du: state = 0;
  Coasting -> (junction 33) : [(throttle >= PedThrs)|(BrkPedDep >= PedThrs)]
  (junction 33) -> drive
  (default) -> drive
  drive -> Coasting : [(throttle < PedThrs)|(BrkPedDep < PedThrs)]
  data: ph_FL input; ph_FR input; ph_RL input; ph_RR input; state output; throttle input; PedThrs input; BrkPedDep input

== stateflow chart S250205simul_switch_2023a/Regen, Tb_max1/Chart ==
  state Coasting
    state OFF
      entry,during:
      YawFlag = 0;
    state ON2
      entry,during:
      YawFlag = 2;
    state ON1
      entry,during:
      YawFlag = 1;
    (default) -> OFF
    OFF -> (junction 46) : [(SASAngle > SASthrs) && (rd_r > Yawthrs)]
    (junction 46) -> ON2
    ON2 -> OFF [order 2] : [(state~=1)&&(rd_r <=Yawthrs)]
    ON1 -> OFF [order 1] : [(MotCoastFrntTq - MotTqCmdFrntVal > -5) && (MotCoastFrntTq - MotTqCmdFrntVal < 5) && (MotCoastRearTq - MotTqCmdRearVal > -5) && (MotCoastRearTq - MotTqCmdRearVal < 5)]
    ON1 -> ON2 [order 2] : [(state~=1)]
    ON2 -> ON1 [order 1] : [(state==1)&&(rd_r <= Yawthrs)]
  state Drive
    en,du:
    YawFlag = 0;
  (default) -> Drive
  Drive -> Coasting : [(PedDep < PedDepthrs)&&(BrkPed < PedDepthrs)]
  Coasting -> Drive : [(PedDep >= PedDepthrs)|(BrkPed >= PedDepthrs)]
  data: rd_r input; PedDep input; SASAngle input; YawFlag output size=1; PedDepthrs input; SASthrs input; Yawthrs input; BrkPed input; MotTqCmdRearVal input; MotTqCmdFrntVal input; MotCoastFrntTq input; MotCoastRearTq input; state input

== stateflow chart S250205simul_switch_2023a/SlipCtrlFL/VmcRgn_Chart ==
  state LSC_On
    state Phase6
      entry,during:
      phase = 6;
    state Phase1
      entry,during:
      phase = 1;
    state Phase2
      entry,during:
      phase = 2;
    state Phase3
      entry,during:
      phase = 3;
    state Phase4
      entry,during:
      phase = 4;
    state Phase5
      entry,during:
      phase = 5;
    Phase6 -> (junction 225) [order 1] : [(yaw_flag == 2)]
    Phase6 -> (junction 235) [order 2] : [(slip > k_6to2*slip_max)]
    (junction 225) -> Phase1
    (junction 235) -> (junction 167)
    Phase2 -> Phase6 [order 1] : [(slip_pred < k_2to6*slip_max)]
    (default) -> Phase1
    Phase1 -> Phase2 : [(slip_pred > k_1to2*slip_max)]
    (junction 167) -> Phase2
    (junction 165) -> (junction 167)
    (junction 217) -> Phase1
    Phase2 -> Phase3 [order 2] : [(slip > k_2to3*slip_max)]
    Phase3 -> Phase4 : [(slip < k_3to4*slip_max)]
    Phase4 -> (junction 217) [order 1] : [(tq_cmd < tq_in)]
    (junction 220) -> (junction 217)
    Phase4 -> Phase5 [order 2] : [(sgn > 0)]
    Phase5 -> (junction 220) [order 1] : [(tq_cmd < tq_in)]
    Phase5 -> (junction 165) [order 2] : [(slip_pred > k_5to2*slip_max)]
  state LSC_off
    entry,during:
    phase = 0;
  state ready
    en, du: phase = 0;
  LSC_On -> (junction 231) : [(PedDep >= PedDep_thrs)]
  (junction 231) -> ready
  (default) -> ready
  LSC_off -> LSC_On : [(sgn > 0)&&(slip > 0)&&(a_car < 0)]
  ready -> LSC_off : [(PedDep < PedDep_thrs)]
  data: phase output; slip input; a_car input; PedDep input; slip_pred input; slip_max input; tq_cmd input; tq_in input; sgn input; yaw_flag input; PedDep_thrs input; k_1to2 input; k_2to3 input; k_2to6 input; k_3to4 input; k_5to2 input; k_6to2 input

== stateflow chart S250205simul_switch_2023a/SlipCtrlFR/VmcRgn_Chart2 ==
  state LSC_On
    state Phase6
      entry,during:
      phase = 6;
    state Phase1
      entry,during:
      phase = 1;
    state Phase2
      entry,during:
      phase = 2;
    state Phase3
      entry,during:
      phase = 3;
    state Phase4
      entry,during:
      phase = 4;
    state Phase5
      entry,during:
      phase = 5;
    Phase6 -> (junction 225) [order 1] : [(yaw_flag == 2)]
    Phase6 -> (junction 235) [order 2] : [(slip > k_6to2*slip_max)]
    (junction 225) -> Phase1
    (junction 235) -> (junction 167)
    Phase2 -> Phase6 [order 1] : [(slip_pred < k_2to6*slip_max)]
    (default) -> Phase1
    Phase1 -> Phase2 : [(slip_pred > k_1to2*slip_max)]
    (junction 167) -> Phase2
    (junction 165) -> (junction 167)
    (junction 217) -> Phase1
    Phase2 -> Phase3 [order 2] : [(slip > k_2to3*slip_max)]
    Phase3 -> Phase4 : [(slip < k_3to4*slip_max)]
    Phase4 -> (junction 217) [order 1] : [(tq_cmd < tq_in)]
    (junction 220) -> (junction 217)
    Phase4 -> Phase5 [order 2] : [(sgn > 0)]
    Phase5 -> (junction 220) [order 1] : [(tq_cmd < tq_in)]
    Phase5 -> (junction 165) [order 2] : [(slip_pred > k_5to2*slip_max)]
  state LSC_off
    entry,during:
    phase = 0;
  state ready
    en, du: phase = 0;
  LSC_On -> (junction 231) : [(PedDep >= PedDep_thrs)]
  (junction 231) -> ready
  (default) -> ready
  LSC_off -> LSC_On : [(sgn > 0)&&(slip > 0)&&(a_car < 0)]
  ready -> LSC_off : [(PedDep < PedDep_thrs)]
  data: phase output; slip input; a_car input; PedDep input; slip_pred input; slip_max input; tq_cmd input; tq_in input; sgn input; yaw_flag input; PedDep_thrs input; k_1to2 input; k_2to3 input; k_2to6 input; k_3to4 input; k_5to2 input; k_6to2 input

== stateflow chart S250205simul_switch_2023a/SlipCtrlRL/VmcRgn_Chart3 ==
  state LSC_On
    state Phase6
      entry,during:
      phase = 6;
    state Phase1
      entry,during:
      phase = 1;
    state Phase2
      entry,during:
      phase = 2;
    state Phase3
      entry,during:
      phase = 3;
    state Phase4
      entry,during:
      phase = 4;
    state Phase5
      entry,during:
      phase = 5;
    Phase6 -> (junction 225) [order 1] : [(yaw_flag == 2)|(tq_cmd < tq_in)]
    Phase6 -> (junction 235) [order 2] : [(slip > k_6to2*slip_max)]
    (junction 225) -> Phase1
    (junction 235) -> (junction 167)
    Phase2 -> Phase6 [order 1] : [(slip_pred < k_2to6*slip_max)]
    (default) -> Phase1
    Phase1 -> Phase2 : [(slip_pred > k_1to2*slip_max)]
    (junction 167) -> Phase2
    (junction 165) -> (junction 167)
    (junction 217) -> Phase1
    Phase2 -> Phase3 [order 2] : [(slip > k_2to3*slip_max)]
    Phase3 -> Phase4 : [(slip < k_3to4*slip_max)]
    Phase4 -> (junction 217) [order 1] : [(tq_cmd < tq_in)]
    (junction 220) -> (junction 217)
    Phase4 -> Phase5 [order 2] : [(sgn > 0)]
    Phase5 -> (junction 220) [order 1] : [(tq_cmd < tq_in)]
    Phase5 -> (junction 165) [order 2] : [(slip_pred > k_5to2*slip_max)]
  state LSC_off
    entry,during:
    phase = 0;
  state ready
    en, du: phase = 0;
  LSC_On -> (junction 231) : [(PedDep >= PedDep_thrs)]
  (junction 231) -> ready
  (default) -> ready
  LSC_off -> LSC_On : [(sgn > 0)&&(slip > 0)&&(a_car < 0)]
  ready -> LSC_off : [(PedDep < PedDep_thrs)]
  data: phase output; slip input; a_car input; PedDep input; slip_pred input; slip_max input; tq_cmd input; tq_in input; sgn input; yaw_flag input; PedDep_thrs input; k_1to2 input; k_2to3 input; k_2to6 input; k_3to4 input; k_5to2 input; k_6to2 input

== stateflow chart S250205simul_switch_2023a/SlipCtrlRR/VmcRgn_Chart4 ==
  state LSC_On
    state Phase6
      entry,during:
      phase = 6;
    state Phase1
      entry,during:
      phase = 1;
    state Phase2
      entry,during:
      phase = 2;
    state Phase3
      entry,during:
      phase = 3;
    state Phase4
      entry,during:
      phase = 4;
    state Phase5
      entry,during:
      phase = 5;
    Phase6 -> (junction 225) [order 1] : [(yaw_flag == 2)]
    Phase6 -> (junction 235) [order 2] : [(slip > k_6to2*slip_max)]
    (junction 225) -> Phase1
    (junction 235) -> (junction 167)
    Phase2 -> Phase6 [order 1] : [(slip_pred < k_2to6*slip_max)]
    (default) -> Phase1
    Phase1 -> Phase2 : [(slip_pred > k_1to2*slip_max)]
    (junction 167) -> Phase2
    (junction 165) -> (junction 167)
    (junction 217) -> Phase1
    Phase2 -> Phase3 [order 2] : [(slip > k_2to3*slip_max)]
    Phase3 -> Phase4 : [(slip < k_3to4*slip_max)]
    Phase4 -> (junction 217) [order 1] : [(tq_cmd < tq_in)]
    (junction 220) -> (junction 217)
    Phase4 -> Phase5 [order 2] : [(sgn > 0)]
    Phase5 -> (junction 220) [order 1] : [(tq_cmd < tq_in)]
    Phase5 -> (junction 165) [order 2] : [(slip_pred > k_5to2*slip_max)]
  state LSC_off
    entry,during:
    phase = 0;
  state ready
    en, du: phase = 0;
  LSC_On -> (junction 231) : [(PedDep >= PedDep_thrs)]
  (junction 231) -> ready
  (default) -> ready
  LSC_off -> LSC_On : [(sgn > 0)&&(slip>0)&&(a_car < 0)]
  ready -> LSC_off : [(PedDep < PedDep_thrs)]
  data: phase output; slip input; a_car input; PedDep input; slip_pred input; slip_max input; tq_cmd input; tq_in input; sgn input; yaw_flag input; PedDep_thrs input; k_1to2 input; k_2to3 input; k_2to6 input; k_3to4 input; k_5to2 input; k_6to2 input
